simulink model "SimPart1"  (R2023b)
settings: Solver=VariableStepAuto  StartTime=0.0  StopTime=2  RelTol=1e-3
values from neighbouring files (symbols this model uses):
  delay = mic_src_d ./ speed    [CompleteSim.m]    (also in SimInitialScript.m; SimMain.m; Simulation.mat = [0.00105053794338 0.00123616464763 0.00169894580427 0.001569)
  fs = 2000    [SimMain.m]    (also in Simulation.mat)
  samplef = (2.5 * fs)    [CompleteSim.m]    (also in SimInitialScript.m; SimMain.m = 5000; Simulation.mat = 5000)
libraries: simulink x1
settings Model: Creator=megan  LastModifiedBy=megan

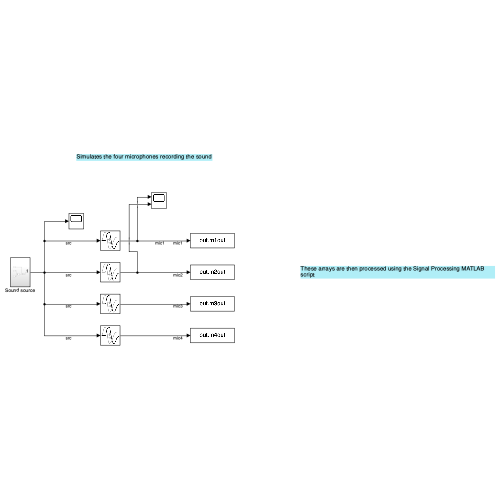
[thumbnail: Simulink's stored preview of the top-level diagram]
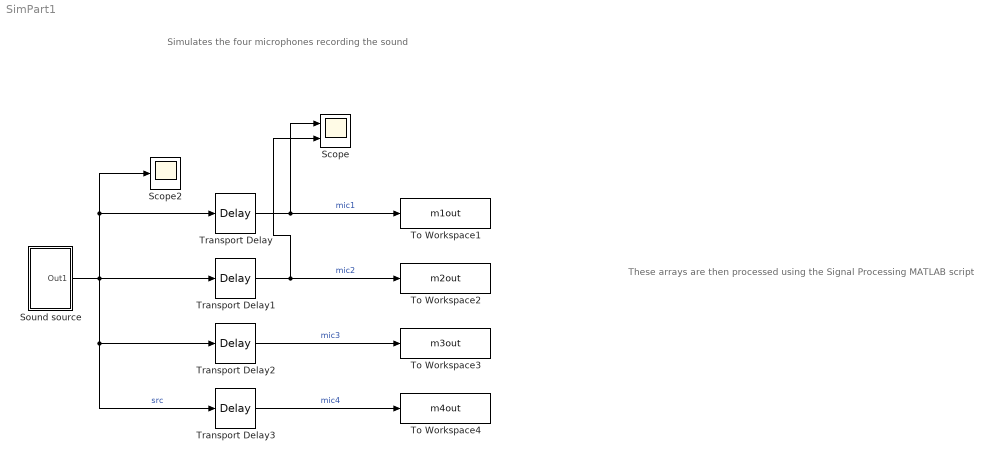
== system SimPart1 ==
  note: Simulates the four microphones recording the sound
  note: These arrays are then processed using the Signal Processing MATLAB script
  Scope : Scope  NumInputPorts=2
  Scope2 : Scope
  Sound source : Subsystem
  To Workspace1 : ToWorkspace  VariableName=m1out  SampleTime=1/samplef
      settings: Save2DSignal=2-D array (concatenate along first dimension)
  To Workspace2 : ToWorkspace  VariableName=m2out  SampleTime=1/samplef
      settings: Save2DSignal=2-D array (concatenate along first dimension)
  To Workspace3 : ToWorkspace  VariableName=m3out  SampleTime=1/samplef
      settings: Save2DSignal=2-D array (concatenate along first dimension)
  To Workspace4 : ToWorkspace  VariableName=m4out  SampleTime=1/samplef
      settings: Save2DSignal=2-D array (concatenate along first dimension)
  Transport Delay : TransportDelay  DelayTime=delay(1)  FixedBuffer=on
  Transport Delay1 : TransportDelay  DelayTime=delay(2)  FixedBuffer=on  TransDelayFeedthrough=on
  Transport Delay2 : TransportDelay  DelayTime=delay(3)  FixedBuffer=on  TransDelayFeedthrough=on
  Transport Delay3 : TransportDelay  DelayTime=delay(4)  FixedBuffer=on  TransDelayFeedthrough=on
  wires:
  Sound source/1(Out1) -> Transport Delay3/1, Transport Delay2/1, Scope2/1, Transport Delay/1, Transport Delay1/1  "src"
  Transport Delay/1 -> Scope/1, To Workspace1/1  "mic1"
  Transport Delay1/1 -> To Workspace2/1, Scope/2  "mic2"
  Transport Delay2/1 -> To Workspace3/1  "mic3"
  Transport Delay3/1 -> To Workspace4/1  "mic4"

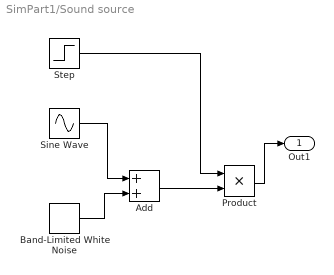
== system SimPart1/Sound source ==
  Add : Sum
  Band-Limited White Noise : simulink/Sources/Band-Limited White Noise  Cov=0.001  Ts=1/samplef  seed=23341
  Product : Product
  Sine Wave : Sin  Amplitude=10  Frequency=fs  SampleTime=1/samplef
  Step : Step  Before=1  After=0  OutDataTypeStr=Inherit: Inherit via back propagation  SampleTime=1/samplef
  Out1 : Outport
  wires:
  Band-Limited White Noise/1 -> Add/2
  Sine Wave/1 -> Add/1
  Step/1 -> Product/1
  Product/1 -> Out1/1
  Add/1 -> Product/2
